simulink model "uz_plantModel_pt1"  (R2020b)
settings: Solver=FixedStepAuto  StartTime=0.0  StopTime=20  RelTol=1e-3
settings Model: DataTypeOverride=Off  Creator=ts  LastModifiedBy=ts
settings DataIOCC: LimitDataPoints=on  SaveOutput=off  SaveTime=off
settings OptimizationCC: BlockReduction=off  ConditionallyExecuteInputs=off  DefaultParameterBehavior=Inlined  LifeSpan=inf
settings DebuggingCC: AlgebraicLoopMsg=error  SingleTaskRateTransMsg=error  AllowSymbolicDim=off  StrictBusMsg=ErrorOnBusTreatedAsVector  SFUnexpectedBacktrackingDiag=warning  SFNoUnconditionalDefaultTransitionDiag=warning  SFExecutionAtInitializationDiag=none  ArithmeticOperatorsInVariantConditions=warning
settings HardwareCC: ProdBitPerPointer=32  ProdBitPerSizeT=32  ProdBitPerPtrDiffT=32  ProdLargestAtomicFloat=None  ProdIntDivRoundTo=Undefined  ProdEndianess=Unspecified  ProdWordSize=32  ProdHWDeviceType=ASIC/FPGA->ASIC/FPGA  ProdEqTarget=off
settings SFSimCC: SimUseLocalCustomCode=off  CustomCodeUndefinedFunction=UseInterfaceOnly
settings RTWCC: RTWUseLocalCustomCode=off
settings CodeAppCC: StateflowObjectComments=on
settings GRTTargetCC: TargetLangStandard=C89/C90 (ANSI)
settings ConfigComp: CovScope=ReferencedModels  CovMetricSettings=dw  CovSaveCumulativeToWorkspaceVar=on  CovSaveSingleToWorkspaceVar=on  CovExternalEMLEnable=off  CovSFcnEnable=off

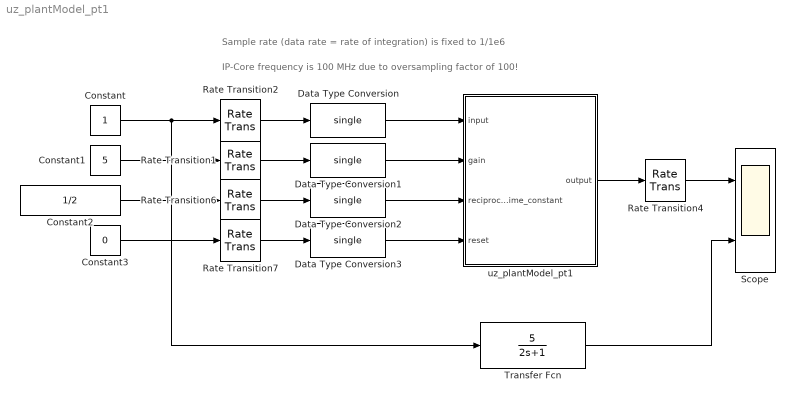
== system uz_plantModel_pt1 ==
  note: IP-Core frequency is 100 MHz due to oversampling factor of 100!
  note: Sample rate (data rate = rate of integration) is fixed to 1/1e6
  Constant : Constant
  Constant1 : Constant  Value=5
  Constant2 : Constant  Value=1/2
  Constant3 : Constant  Value=0
  Data Type Conversion{,1..3} (4 alike) : DataTypeConversion  OutDataTypeStr=single
  Rate Transition{1..2,6..7} (4 alike) : RateTransition  OutPortSampleTime=1/1e6
  Rate Transition4 : RateTransition
  Scope : Scope  NumInputPorts=2
  Transfer Fcn : TransferFcn  Numerator=[5]  Denominator=[2 1]
  uz_plantModel_pt1 : Subsystem  TreatAsAtomicUnit=on
  wires:
  uz_plantModel_pt1/1(output) -> Rate Transition4/1
  Constant/1 -> Rate Transition2/1, Transfer Fcn/1
  Rate Transition4/1 -> Scope/1
  Transfer Fcn/1 -> Scope/2
  Rate Transition2/1 -> Data Type Conversion/1
  Data Type Conversion/1 -> uz_plantModel_pt1/1(input)
  Data Type Conversion1/1 -> uz_plantModel_pt1/2(gain)
  Data Type Conversion2/1 -> uz_plantModel_pt1/3(reciprocal_time_constant)
  Data Type Conversion3/1 -> uz_plantModel_pt1/4(reset)
  Rate Transition1/1 -> Data Type Conversion1/1
  Rate Transition6/1 -> Data Type Conversion2/1
  Rate Transition7/1 -> Data Type Conversion3/1
  Constant1/1 -> Rate Transition1/1
  Constant2/1 -> Rate Transition6/1
  Constant3/1 -> Rate Transition7/1

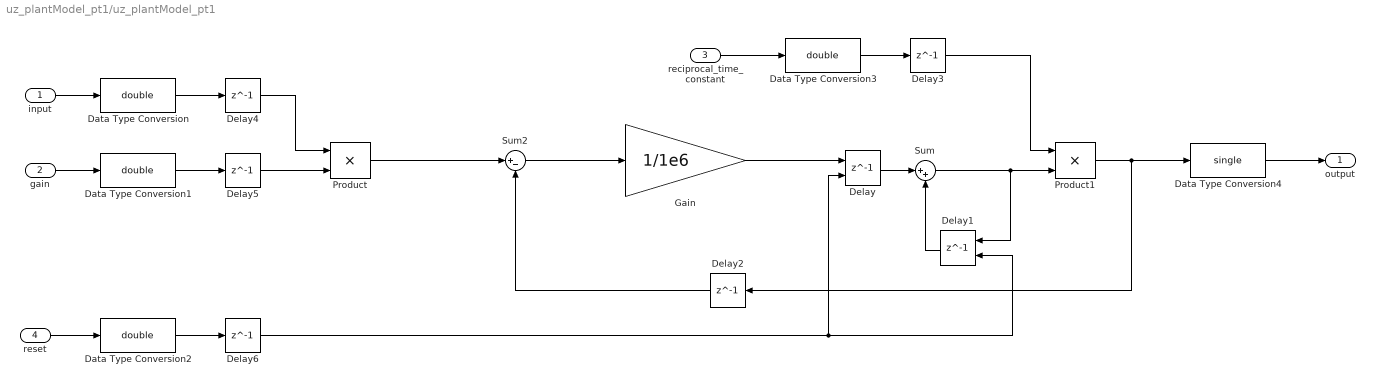
== system uz_plantModel_pt1/uz_plantModel_pt1 ==
  input : Inport
  gain : Inport  Port=2
  reciprocal_time_constant : Inport  Port=3
  reset : Inport  Port=4
  Data Type Conversion{,1..3} (4 alike) : DataTypeConversion  OutDataTypeStr=double  RndMeth=Nearest
  Data Type Conversion4 : DataTypeConversion  OutDataTypeStr=single  RndMeth=Nearest
  Delay : Delay  DelayLength=1  ExternalReset=Level
      settings: InputPortMap=u0,r5
  Delay1 : Delay  DelayLength=1  ExternalReset=Level
      settings: InputPortMap=u0,r5
  Delay{2..6} (5 alike) : Delay  DelayLength=1
  Gain : Gain  Gain=1/1e6  OutDataTypeStr=double
  Product : Product
  Product1 : Product
  Sum : Sum  Inputs=|++  OutDataTypeStr=double
  Sum2 : Sum  Inputs=|+-
  output : Outport
  wires:
  Sum/1 -> Product1/2, Delay1/1
  Delay4/1 -> Product/1
  Delay5/1 -> Product/2
  reciprocal_time_constant/1 -> Data Type Conversion3/1
  Delay/1 -> Sum/1
  Delay1/1 -> Sum/2
  Gain/1 -> Delay/1
  reset/1 -> Data Type Conversion2/1
  Delay3/1 -> Product1/1
  input/1 -> Data Type Conversion/1
  gain/1 -> Data Type Conversion1/1
  Delay6/1 -> Delay1/2, Delay/2
  Sum2/1 -> Gain/1
  Delay2/1 -> Sum2/2
  Product/1 -> Sum2/1
  Product1/1 -> Data Type Conversion4/1, Delay2/1
  Data Type Conversion/1 -> Delay4/1
  Data Type Conversion1/1 -> Delay5/1
  Data Type Conversion2/1 -> Delay6/1
  Data Type Conversion3/1 -> Delay3/1
  Data Type Conversion4/1 -> output/1
